simulink model "si4_springmass_damper"  (R2024a)
settings: Solver=VariableStepAuto  StartTime=0.0  StopTime=te  RelTol=1e-3  EnableMultiTasking=on
values from neighbouring files (symbols this model uses):
  c = -0.8    [si5_Ball_parameter.m]    (also in sim21_ODE.m = 1)
  k = 10    [si5_Ball_parameter.m]    (also in sim21_ODE.m = 3)
  m = 0.35    [Electromagnet_par.m]    (also in si5_Ball_parameter.m = 0.1; sim21_ODE.m = 3)
  x0 = 0.01    [Electromagnet_par.m]    (also in sim21_ODE.m = [0 0])
settings Model: Creator=sar  LastModifiedBy=ocean
settings SolverCC: AlgebraicLoopSolver=TrustRegion
settings DataIOCC: LimitDataPoints=on  ReturnWorkspaceOutputs=off  Refine=10
settings OptimizationCC: LifeSpan=inf
settings DebuggingCC: UnconnectedInputMsg=warning  UnconnectedOutputMsg=warning  UnconnectedLineMsg=warning  AllowSymbolicDim=off  SFUnexpectedBacktrackingDiag=warning  SFNoUnconditionalDefaultTransitionDiag=warning  SFExecutionAtInitializationDiag=none  ArithmeticOperatorsInVariantConditions=warning
settings ModelReferenceCC: EnableRefExpFcnMdlSchedulingChecks=on  PropagateSignalLabelsOutOfModel=off
settings SFSimCC: SimUseLocalCustomCode=off  CustomCodeUndefinedFunction=UseInterfaceOnly
settings RTWCC: RTWUseLocalCustomCode=off  GPUComputeCapability=3.5  DLArmComputeVersion=19.05
settings CodeAppCC: StateflowObjectComments=on
settings GRTTargetCC: TargetLangStandard=C89/C90 (ANSI)
settings ConfigComp: CovMetricSettings=dw  CovSaveCumulativeToWorkspaceVar=on  CovSaveSingleToWorkspaceVar=on  CovExternalEMLEnable=off

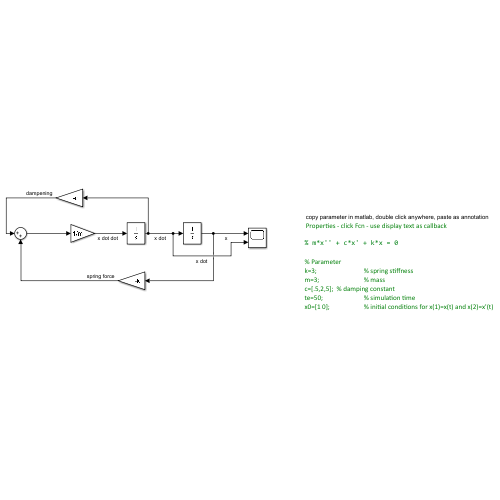
[thumbnail: Simulink's stored preview of the top-level diagram]
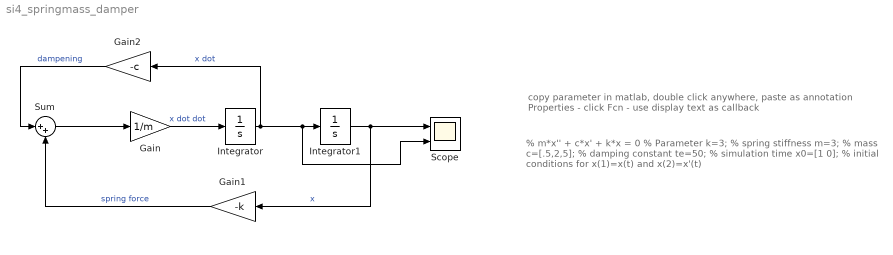
== system si4_springmass_damper ==
  note: copy parameter in matlab, double click anywhere, paste as annotation
      | Properties - click Fcn - use display text as callback
  note: % m*x'' + c*x' + k*x = 0
      |
      | % Parameter
      | k=3; % spring stiffness
      | m=3; % mass
      | c=[.5,2,5]; % damping constant
      | te=50; % simulation time
      | x0=[1 0]; % initial conditions for x(1)=x(t) and x(2)=x'(t)
  Gain : Gain  Gain=1/m
  Gain1 : Gain  Gain=-k
  Gain2 : Gain  Gain=-c
  Integrator : Integrator  InitialCondition=x0(2)
  Integrator1 : Integrator  InitialCondition=x0(1)
  Scope : Scope  NumInputPorts=2
  Sum : Sum  Inputs=|++
  wires:
  Gain/1 -> Integrator/1  "x dot dot"
  Integrator/1 -> Gain2/1, Scope/2, Integrator1/1  "x dot"
  Integrator1/1 -> Gain1/1, Scope/1  "x"
  Gain1/1 -> Sum/2  "spring force"
  Gain2/1 -> Sum/1  "dampening"
  Sum/1 -> Gain/1
